simulink model "testControlWithDroneSwarm_r2021b"  (R2021b)
settings: Solver=ode4  StartTime=0.0  StopTime=inf  FixedStep=sample_time_base  RelTol=1e-3
InitFcn:
  | init_condition();
StopFcn:
  | stop_function();
values from neighbouring files (symbols this model uses):
  activate_sim = true    [init_condition.m]
  local_ip = param_simulink.local_ip    [init_condition.m]
  local_ip_sim = param_simulink.local_ip    [init_condition.m]
  number = params.number    [init_condition.m]    (also in visualization.m = size(position0,2))
  number_real = min(param_simulink.number_real,number)    [init_condition.m]    (also in visualization.m = mat_file.number_real)
  number_sim = max(number - number_real,0)    [init_condition.m]
  position0_sim = position0(:,number-number_sim+1:end)    [init_condition.m]
  sample_time_base = 0.0025    [init_condition.m]
  sample_time_control_bottom = sample_time_control_upper    [init_condition.m]
  sample_time_control_upper = params.sample_time_control_upper    [init_condition.m]
  sample_time_motion = sample_time_control_upper    [init_condition.m]    (also in visualization.m = mat_file.sample_time_base)
  target_ip_array = param_simulink.target_ip    [init_condition.m]
  target_ip_array_sim = param_simulink.target_ip(number-number_sim+1:number)    [init_condition.m]
undefined symbols (not defined in the file or in its folder): get_array_slice, map3d_faces, map3d_struct, position0
libraries: aerolibanimutils x1, dspindex x1
settings Model: Creator=huangjialei  LastModifiedBy=Huang Jialei

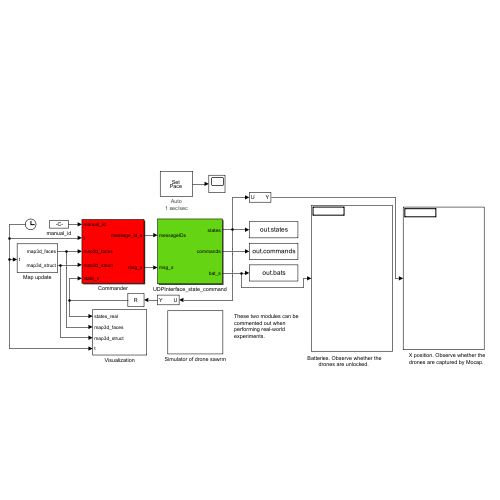
[thumbnail: Simulink's stored preview of the top-level diagram]
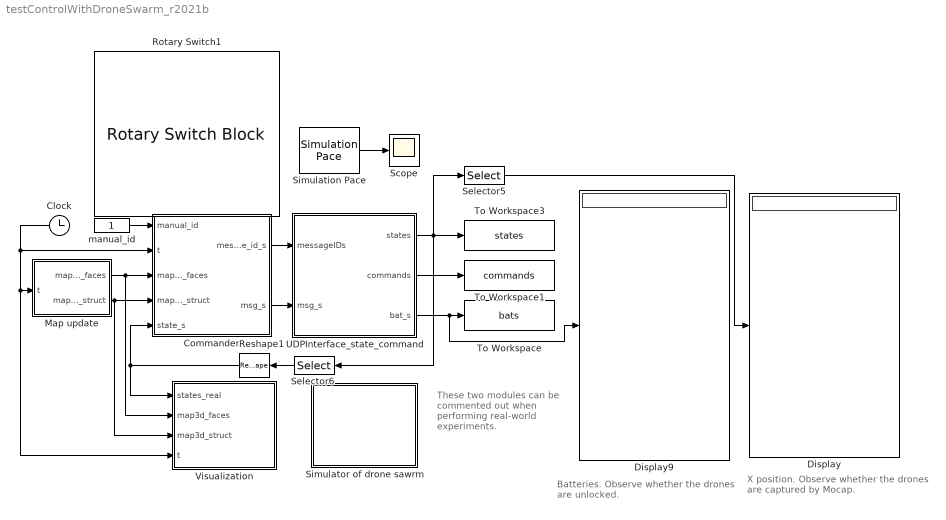
== system testControlWithDroneSwarm_r2021b ==
  note: These two modules can be commented out when performing real-world experiments.
  note: Batteries. Observe whether the drones are unlocked.
  note: X position. Observe whether the drones are captured by Mocap.
  Clock : Clock
  Commander : Subsystem
  Display : Display
  Display9 : Display
  Map update : Subsystem
  Reshape1 : Reshape  OutputDimensionality=Customize  OutputDimensions=[12,number]
  Rotary Switch1 : RotarySwitchBlock
      settings: Values={{'Arming', 'Takeoff', 'Hover', 'Land', 'Alg', 'Test', 'None'}, [1 2 3 4 5 6 1111]}
  Scope : Scope
  Selector5 : Selector  InputPortWidth=17*number  IndexOptions=Index vector (dialog)  Indices=get_array_slice([1,6], number, 17)  OutputSizes=1
  Selector6 : Selector  InputPortWidth=17*number  IndexOptions=Index vector (dialog)  Indices=get_array_slice(6:17, number, 17)  OutputSizes=1
  Simulation Pace : aerolibanimutils/Simulation Pace  SimulationPace=1  SleepMode=Auto  OutputPaceError=on  SampleTime=sample_time_base
  Simulator of drone sawrm : Subsystem
  To Workspace : ToWorkspace  VariableName=bats  SaveFormat=Timeseries  SampleTime=-1
  To Workspace1 : ToWorkspace  VariableName=commands  SaveFormat=Timeseries  SampleTime=-1
  To Workspace3 : ToWorkspace  VariableName=states  SaveFormat=Timeseries  SampleTime=-1
  UDPInterface_state_command : Subsystem
  Visualization : Subsystem
  manual_id : Constant
  wires:
  UDPInterface_state_command/1(states) -> Selector6/1, To Workspace3/1, Selector5/1
  Commander/2(msg_s) -> UDPInterface_state_command/2(msg_s)
  UDPInterface_state_command/2(commands) -> To Workspace1/1
  Commander/1(message_id_s) -> UDPInterface_state_command/1(messageIDs)
  UDPInterface_state_command/3(bat_s) -> Display9/1, To Workspace/1
  Selector5/1 -> Display/1
  manual_id/1 -> Commander/1(manual_id)
  Selector6/1 -> Reshape1/1
  Reshape1/1 -> Commander/5(state_s), Visualization/1(states_real)
  Simulation Pace/1 -> Scope/1
  Map update/1(map3d_faces) -> Visualization/2(map3d_faces), Commander/3(map3d_faces)
  Map update/2(map3d_struct) -> Visualization/3(map3d_struct), Commander/4(map3d_struct)
  Clock/1 -> Visualization/4(t), Map update/1(t), Commander/2(t)

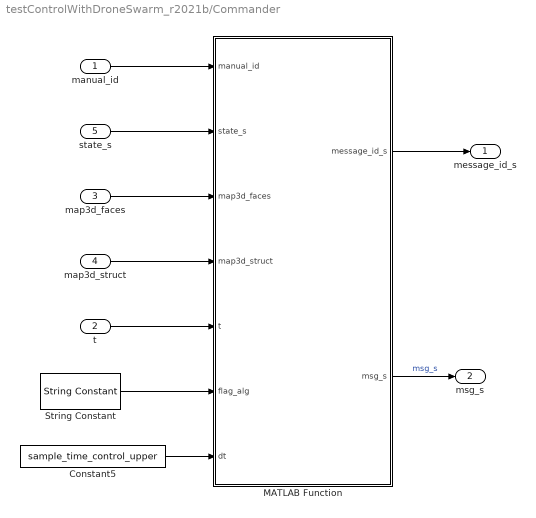
== system testControlWithDroneSwarm_r2021b/Commander ==
  manual_id : Inport
  t : Inport  Port=2
  map3d_faces : Inport  Port=3
  map3d_struct : Inport  Port=4
  state_s : Inport  Port=5
  Constant5 : Constant  Value=sample_time_control_upper
  MATLAB Function : MATLAB Function  TreatAsAtomicUnit=on  SystemSampleTime=sample_time_control_upper
  String Constant : StringConstant  String=flag_alg
  message_id_s : Outport
  msg_s : Outport  Port=2
  wires:
  MATLAB Function/2(msg_s) -> msg_s/1  "msg_s"
  manual_id/1 -> MATLAB Function/1(manual_id)
  t/1 -> MATLAB Function/5(t)
  map3d_faces/1 -> MATLAB Function/3(map3d_faces)
  map3d_struct/1 -> MATLAB Function/4(map3d_struct)
  MATLAB Function/1(message_id_s) -> message_id_s/1
  String Constant/1 -> MATLAB Function/6(flag_alg)
  Constant5/1 -> MATLAB Function/7(dt)
  state_s/1 -> MATLAB Function/2(state_s)

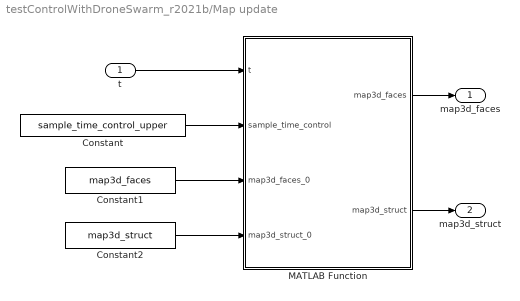
== system testControlWithDroneSwarm_r2021b/Map update ==
  t : Inport
  Constant : Constant  Value=sample_time_control_upper
  Constant1 : Constant  Value=map3d_faces
  Constant2 : Constant  Value=map3d_struct
  MATLAB Function : MATLAB Function  TreatAsAtomicUnit=on  SystemSampleTime=sample_time_control_upper
  map3d_faces : Outport
  map3d_struct : Outport  Port=2
  wires:
  MATLAB Function/1(map3d_faces) -> map3d_faces/1
  MATLAB Function/2(map3d_struct) -> map3d_struct/1
  t/1 -> MATLAB Function/1(t)
  Constant/1 -> MATLAB Function/2(sample_time_control)
  Constant1/1 -> MATLAB Function/3(map3d_faces_0)
  Constant2/1 -> MATLAB Function/4(map3d_struct_0)

== system testControlWithDroneSwarm_r2021b/Simulator of drone sawrm ==
  Constant : Constant  Value=activate_sim
  Simulation : Subsystem
  wires:
  Constant/1 -> Simulation/Enable

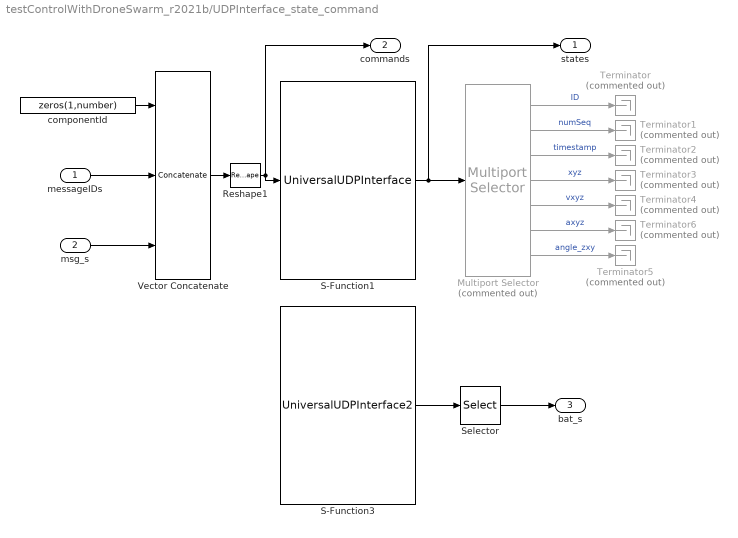
== system testControlWithDroneSwarm_r2021b/UDPInterface_state_command ==
  messageIDs : Inport
  msg_s : Inport  Port=2
  Multiport Selector : dspindex/Multiport Selector  Commented=on  rowsOrCols=Rows  idxCellArray={1:15:15*number,2:15:15*number,3:15:15*number,repmat(4:6,1,number) + reshape(repmat((0:number-1)*15,3,1),1,3*number), repmat(7:9,1,number) + reshape(repmat((0:number-1)*15,3,1),1,3*number), repmat(10:12,1,number) + reshape(repmat((0:number-1)*15,3,1),1,3*number), repmat(13:15,1,number) + reshape(repmat((0:number-1)*15,3,1),1,3*number)}  idxErrMode=Clip Index
  Reshape1 : Reshape
  S-Function1 : S-Function  FunctionName=UniversalUDPInterface  Parameters=sampleTime,number,portTarget,portLocal,ipTarget,ipLocal,flagSend,flagRecv,inputPortWidth,outputPortWidth  SFunctionDeploymentMode=off  EnableBusSupport=off  mask{number=number, ipLocal=local_ip, ipTarget=target_ip_array, portTarget=21000, portLocal=21000, flagSend=on, flagRecv=on, inputPortWidth=6, outputPortWidth=17, sampleTime=sample_time_control_upper}
      mask prompts: number "Number of vehicles"; ipLocal "Local ip"; ipTarget "Target ip"; portTarget "Start port of target"; portLocal "Start port of local"; flagSend "Enable sender"; flagRecv "Enable receiver"; inputPortWidth "Width of input port"; outputPortWidth "Width of output port"; sampleTime "Sample time"
      mask help:
      | input port: componentId, messageId, msgData[0], msgData[1], ...
      | output port: systemId, numSequence, timeStamp,msgData[0], msgData[1], ...
  S-Function3 : S-Function  FunctionName=UniversalUDPInterface2  Parameters=sampleTime,number,portTarget,portLocal,ipTarget,ipLocal,flagSend,flagRecv,inputPortWidth,outputPortWidth  SFunctionDeploymentMode=off  EnableBusSupport=off  mask{number=number, ipLocal=local_ip, ipTarget=target_ip_array, portTarget=22000, portLocal=20000, flagSend=off, flagRecv=on, inputPortWidth=3, outputPortWidth=6, sampleTime=sample_time_control_upper}
      mask prompts: number "Number of vehicles"; ipLocal "Local ip"; ipTarget "Target ip"; portTarget "Start port of target"; portLocal "Start port of local"; flagSend "Enable sender"; flagRecv "Enable receiver"; inputPortWidth "Width of input port"; outputPortWidth "Width of output port"; sampleTime "Sample time"
      mask help:
      | input port: componentId, messageId, msgData[0], msgData[1], ...
      | output port: systemId, numSequence, timeStamp,msgData[0], msgData[1], ...
  Selector : Selector  InputPortWidth=6*number  IndexOptions=Index vector (dialog)  Indices=get_array_slice([1,6], number, 6)  OutputSizes=1
  Terminator{,1..6} (7 alike) : Terminator  Commented=on
  Vector Concatenate : Concatenate  NumInputs=3  Mode=Multidimensional array
  componentId : Constant  Value=zeros(1,number)  VectorParams1D=off
  states : Outport
  commands : Outport  Port=2
  bat_s : Outport  Port=3
  wires:
  Multiport Selector/2 -> Terminator1/1  "numSeq"
  Multiport Selector/5 -> Terminator4/1  "vxyz"
  Vector Concatenate/1 -> Reshape1/1
  Multiport Selector/3 -> Terminator2/1  "timestamp"
  messageIDs/1 -> Vector Concatenate/2
  Reshape1/1 -> S-Function1/1, commands/1
  componentId/1 -> Vector Concatenate/1
  Multiport Selector/4 -> Terminator3/1  "xyz"
  Multiport Selector/1 -> Terminator/1  "ID"
  msg_s/1 -> Vector Concatenate/3
  S-Function3/1 -> Selector/1
  Selector/1 -> bat_s/1
  Multiport Selector/7 -> Terminator5/1  "angle_zxy"
  Multiport Selector/6 -> Terminator6/1  "axyz"
  S-Function1/1 -> states/1, Multiport Selector/1

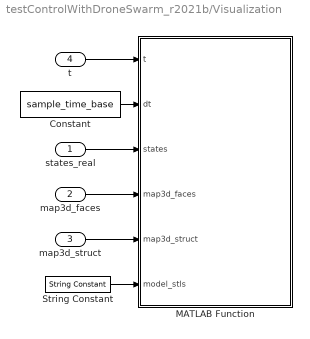
== system testControlWithDroneSwarm_r2021b/Visualization ==
  states_real : Inport
  map3d_faces : Inport  Port=2
  map3d_struct : Inport  Port=3
  t : Inport  Port=4
  Constant : Constant  Value=sample_time_base
  MATLAB Function : MATLAB Function  TreatAsAtomicUnit=on  SystemSampleTime=sample_time_base
  String Constant : StringConstant  String=model_stls
  wires:
  map3d_faces/1 -> MATLAB Function/4(map3d_faces)
  map3d_struct/1 -> MATLAB Function/5(map3d_struct)
  states_real/1 -> MATLAB Function/3(states)
  t/1 -> MATLAB Function/1(t)
  Constant/1 -> MATLAB Function/2(dt)
  String Constant/1 -> MATLAB Function/6(model_stls)

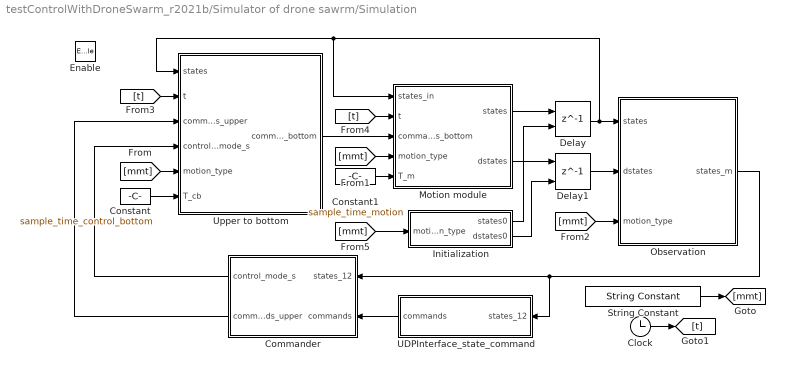
== system testControlWithDroneSwarm_r2021b/Simulator of drone sawrm/Simulation ==
  Enable : EnablePort
  Clock : Clock
  Commander : Subsystem
  Constant : Constant  Value=sample_time_control_bottom
  Constant1 : Constant  Value=sample_time_motion
  Delay : Delay  DelayLength=1  InitialConditionSource=Input port  InitialCondition=0
      settings: InputPortMap=u0,p4
  Delay1 : Delay  DelayLength=1  InitialConditionSource=Input port  InitialCondition=0
      settings: InputPortMap=u0,p4
  Initialization : Subsystem
  Motion module : Subsystem
  Observation : Subsystem
  String Constant : StringConstant  String=motion_model_type
  UDPInterface_state_command : Subsystem
  Upper to bottom : Subsystem
  wires:
  Initialization/2(dstates0) -> Delay1/2
  Delay1/1 -> Observation/2(dstates)
  Motion module/1(states) -> Delay/1
  [mmt] -> Observation/3(motion_type)
  Constant/1 -> Upper to bottom/6(T_cb)
  Upper to bottom/1(commands_bottom) -> Motion module/3(commands_bottom)
  [mmt] -> Motion module/4(motion_type)
  Motion module/2(dstates) -> Delay1/1
  Constant1/1 -> Motion module/5(T_m)
  String Constant/1 -> [mmt]
  UDPInterface_state_command/1(commands) -> Commander/2(commands)
  [mmt] -> Initialization/1(motion_type)
  Commander/1(control_mode_s) -> Upper to bottom/4(control_mode_s)
  Delay/1 -> Observation/1(states), Motion module/1(states_in), Upper to bottom/1(states)
  [t] -> Upper to bottom/2(t)
  Observation/1(states_m) -> Commander/1(states_12), UDPInterface_state_command/1(states_12)
  Initialization/1(states0) -> Delay/2
  [t] -> Motion module/2(t)
  [mmt] -> Upper to bottom/5(motion_type)
  Clock/1 -> [t]
  Commander/2(commands_upper) -> Upper to bottom/3(commands_upper)

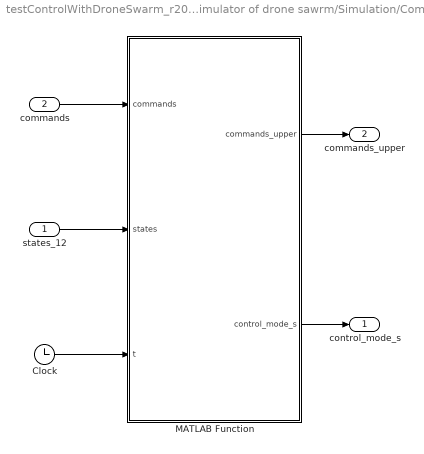
== system testControlWithDroneSwarm_r2021b/Simulator of drone sawrm/Simulation/Commander ==
  states_12 : Inport
  commands : Inport  Port=2
  Clock : Clock
  MATLAB Function : MATLAB Function  TreatAsAtomicUnit=on  SystemSampleTime=sample_time_control_upper
  control_mode_s : Outport
  commands_upper : Outport  Port=2
  wires:
  commands/1 -> MATLAB Function/1(commands)
  states_12/1 -> MATLAB Function/2(states)
  MATLAB Function/1(commands_upper) -> commands_upper/1
  MATLAB Function/2(control_mode_s) -> control_mode_s/1
  Clock/1 -> MATLAB Function/3(t)

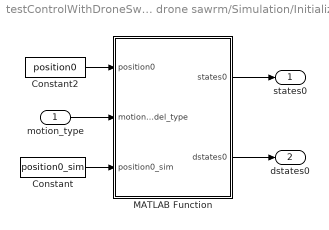
== system testControlWithDroneSwarm_r2021b/Simulator of drone sawrm/Simulation/Initialization ==
  motion_type : Inport
  Constant : Constant  Value=position0_sim
  Constant2 : Constant  Value=position0
  MATLAB Function : MATLAB Function  TreatAsAtomicUnit=on
  states0 : Outport
  dstates0 : Outport  Port=2
  wires:
  MATLAB Function/1(states0) -> states0/1
  Constant2/1 -> MATLAB Function/1(position0)
  motion_type/1 -> MATLAB Function/2(motion_model_type)
  MATLAB Function/2(dstates0) -> dstates0/1
  Constant/1 -> MATLAB Function/3(position0_sim)

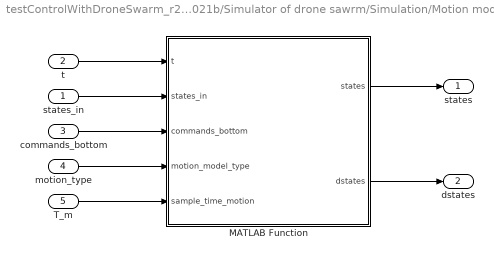
== system testControlWithDroneSwarm_r2021b/Simulator of drone sawrm/Simulation/Motion module ==
  states_in : Inport
  t : Inport  Port=2
  commands_bottom : Inport  Port=3
  motion_type : Inport  Port=4
  T_m : Inport  Port=5
  MATLAB Function : MATLAB Function  TreatAsAtomicUnit=on  SystemSampleTime=sample_time_motion
  states : Outport
  dstates : Outport  Port=2
  wires:
  t/1 -> MATLAB Function/1(t)
  MATLAB Function/1(states) -> states/1
  MATLAB Function/2(dstates) -> dstates/1
  states_in/1 -> MATLAB Function/2(states_in)
  commands_bottom/1 -> MATLAB Function/3(commands_bottom)
  motion_type/1 -> MATLAB Function/4(motion_model_type)
  T_m/1 -> MATLAB Function/5(sample_time_motion)

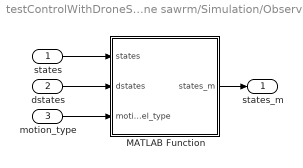
== system testControlWithDroneSwarm_r2021b/Simulator of drone sawrm/Simulation/Observation ==
  states : Inport
  dstates : Inport  Port=2
  motion_type : Inport  Port=3
  MATLAB Function : MATLAB Function  TreatAsAtomicUnit=on
  states_m : Outport
  wires:
  MATLAB Function/1(states_m) -> states_m/1
  states/1 -> MATLAB Function/1(states)
  dstates/1 -> MATLAB Function/2(dstates)
  motion_type/1 -> MATLAB Function/3(motion_model_type)

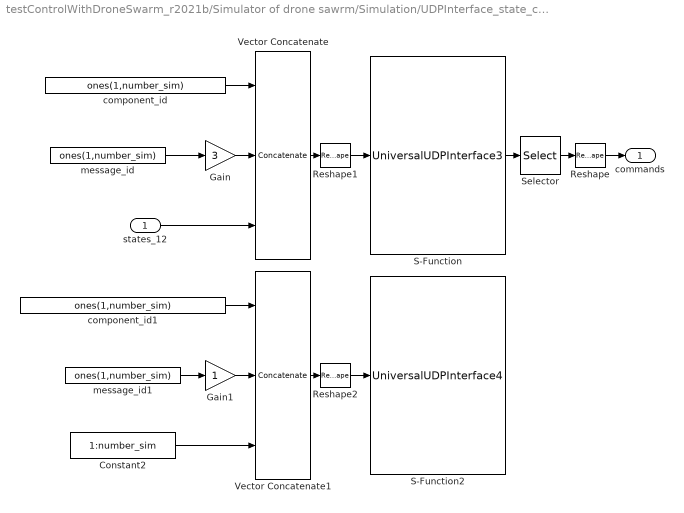
== system testControlWithDroneSwarm_r2021b/Simulator of drone sawrm/Simulation/UDPInterface_state_command ==
  states_12 : Inport
  Constant2 : Constant  Value=1:number_sim  VectorParams1D=off
  Gain : Gain  Gain=3
  Gain1 : Gain
  Reshape : Reshape  OutputDimensionality=Customize  OutputDimensions=[6,number_sim]
  Reshape1 : Reshape
  Reshape2 : Reshape
  S-Function : S-Function  FunctionName=UniversalUDPInterface3  Parameters=sampleTime,number,portTarget,portLocal,ipTarget,ipLocal,flagSend,flagRecv,inputPortWidth,outputPortWidth  SFunctionDeploymentMode=off  EnableBusSupport=off  mask{number=number_sim, ipLocal=local_ip_sim, ipTarget=target_ip_array_sim, portTarget=20999+number_real*2, portLocal=21001+number_real*2, flagSend=on, flagRecv=on, inputPortWidth=14, outputPortWidth=9, sampleTime=sample_time_control_upper}
      mask prompts: number "Number of vehicles"; ipLocal "Local ip"; ipTarget "Target ip"; portTarget "Start port of target"; portLocal "Start port of local"; flagSend "Enable sender"; flagRecv "Enable receiver"; inputPortWidth "Width of input port"; outputPortWidth "Width of output port"; sampleTime "Sample time"
      mask help:
      | input port: componentId, messageId, msgData[0], msgData[1], ...
      | output port: systemId, numSequence, timeStamp,msgData[0], msgData[1], ...
  S-Function2 : S-Function  FunctionName=UniversalUDPInterface4  Parameters=sampleTime,number,portTarget,portLocal,ipTarget,ipLocal,flagSend,flagRecv,inputPortWidth,outputPortWidth  SFunctionDeploymentMode=off  EnableBusSupport=off  mask{number=number_sim, ipLocal=local_ip_sim, ipTarget=target_ip_array_sim, portTarget=19999+number_real*2, portLocal=22001+number_real*2, flagSend=on, flagRecv=off, inputPortWidth=3, outputPortWidth=9, sampleTime=sample_time_control_upper}
      mask prompts: number "Number of vehicles"; ipLocal "Local ip"; ipTarget "Target ip"; portTarget "Start port of target"; portLocal "Start port of local"; flagSend "Enable sender"; flagRecv "Enable receiver"; inputPortWidth "Width of input port"; outputPortWidth "Width of output port"; sampleTime "Sample time"
      mask help:
      | input port: componentId, messageId, msgData[0], msgData[1], ...
      | output port: systemId, numSequence, timeStamp,msgData[0], msgData[1], ...
  Selector : Selector  InputPortWidth=9*number_sim  IndexOptions=Index vector (dialog)  Indices=get_array_slice(4:9, number_sim, 9)  OutputSizes=1
  Vector Concatenate : Concatenate  NumInputs=3  Mode=Multidimensional array
  Vector Concatenate1 : Concatenate  NumInputs=3  Mode=Multidimensional array
  component_id : Constant  Value=ones(1,number_sim)  VectorParams1D=off
  component_id1 : Constant  Value=ones(1,number_sim)  VectorParams1D=off
  message_id : Constant  Value=ones(1,number_sim)  VectorParams1D=off
  message_id1 : Constant  Value=ones(1,number_sim)  VectorParams1D=off
  commands : Outport
  wires:
  Reshape/1 -> commands/1
  Selector/1 -> Reshape/1
  states_12/1 -> Vector Concatenate/3
  Vector Concatenate1/1 -> Reshape2/1
  Reshape2/1 -> S-Function2/1
  component_id1/1 -> Vector Concatenate1/1
  Constant2/1 -> Vector Concatenate1/3
  message_id1/1 -> Gain1/1
  Gain1/1 -> Vector Concatenate1/2
  S-Function/1 -> Selector/1
  Gain/1 -> Vector Concatenate/2
  message_id/1 -> Gain/1
  component_id/1 -> Vector Concatenate/1
  Reshape1/1 -> S-Function/1
  Vector Concatenate/1 -> Reshape1/1

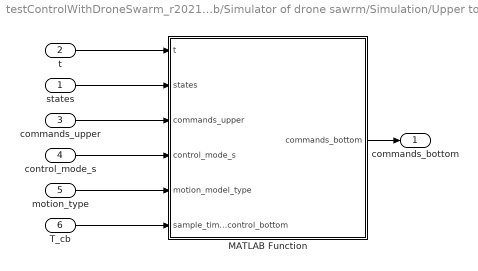
== system testControlWithDroneSwarm_r2021b/Simulator of drone sawrm/Simulation/Upper to bottom ==
  states : Inport
  t : Inport  Port=2
  commands_upper : Inport  Port=3
  control_mode_s : Inport  Port=4
  motion_type : Inport  Port=5
  T_cb : Inport  Port=6
  MATLAB Function : MATLAB Function  TreatAsAtomicUnit=on  SystemSampleTime=sample_time_control_bottom
  commands_bottom : Outport
  wires:
  MATLAB Function/1(commands_bottom) -> commands_bottom/1
  states/1 -> MATLAB Function/2(states)
  t/1 -> MATLAB Function/1(t)
  commands_upper/1 -> MATLAB Function/3(commands_upper)
  control_mode_s/1 -> MATLAB Function/4(control_mode_s)
  motion_type/1 -> MATLAB Function/5(motion_model_type)
  T_cb/1 -> MATLAB Function/6(sample_time_control_bottom)

== matlab function testControlWithDroneSwarm_r2021b/Simulator of drone sawrm/Simulation/Initialization/MATLAB Function ==
  data: position0 input; states0 output; motion_model_type input; dstates0 output; position0_sim input
function [states0,dstates0] = fcn(position0, motion_model_type, position0_sim)

number_sim = size(position0_sim,2);
number = size(position0,2);
states0 = zeros(17,number_sim);
dstates0 = zeros(17,number_sim);

number_real = number - number_sim;

[states,dstates] = initialize_states(position0, motion_model_type);


temp = size(states,1);
states0(1:temp,:) = states(:,number_real+1:end);
temp = size(dstates,1);
dstates0(1:temp,:) = dstates(:,number_real+1:end);

== matlab function testControlWithDroneSwarm_r2021b/Commander/MATLAB Function ==
  data: message_id_s output; manual_id input; state_s input; msg_s output; map3d_faces input; map3d_struct input; t input; flag_alg input; dt input
function [message_id_s, msg_s] = swarm_algorithm(manual_id,state_s, map3d_faces, map3d_struct, t, flag_alg, dt)

number_all = size(state_s,2);
msg_s = zeros(4,number_all);
message_id_s = zeros(1,number_all);

% If the agent is not captured by mocap, its states are all 0. 
is_running = sum(abs(state_s(1:6,:)),1) > 0.001;

%%
% Value of rotary switch
manual_arming = 1;
manual_takeoff = 2;
manual_hover = 3;
manual_land = 4;
manual_alg = 5;
manual_test = 6;
% External control mode
Arming_type = 1;
Takeoff_type = 2;
Hover_type = 3;
Land_type = 4;
Position_control_type = 5;
Velocity_control_type = 6;
Velocity_horizontal_control_type = 7;

% coder.extrinsic('swarm_module_generate_desire');
% coder.extrinsic('py.sorted');
% disp(py.sorted([2,3,1]));
%
h_takeoff = 0.7;
h_land = 0.0;
switch manual_id
    case manual_arming
        message_id_s = Arming_type * ones(1,number_all);
        msg_s = zeros(4,number_all);
    case manual_takeoff
        message_id_s = Takeoff_type * ones(1,number_all);
        msg_s = zeros(4,number_all);
        msg_s(1,:) = h_takeoff;
    case manual_hover
        message_id_s = Hover_type * ones(1,number_all);
        msg_s = zeros(4,number_all);
    case manual_land
        message_id_s = Land_type * ones(1,number_all);
        msg_s = zeros(4,number_all);
        msg_s(1,:) = h_land;
    case manual_alg
        id_is_running = find(is_running);
%         vel_desired = zeros(2, length(id_is_running));
        number_isr = length(id_is_running);
        pos_desired_s_isr = zeros(4,number_isr);
        vel_desired_s_isr = zeros(4,number_isr);

        if sensor_env_module_get_activate()
            motion_model_type = 'quadcopter'; %%%%%%%%%%%%%%%%%%%%
            sensor_data_s = sensor_env_module_get_data_all(state_s(:,id_is_running), motion_model_type, map3d_faces);
        else
            sensor_data_s = [];
        end
        [command_upper_s_isr,control_mode_s_u_isr] = ...
            swarm_module_generate_desire(t, state_s(:,id_is_running), flag_alg, dt, sensor_data_s, map3d_struct);
        
        pos_desired_s_isr(:) = command_upper_s_isr(1:4,1:number_isr);
        vel_desired_s_isr(:) = command_upper_s_isr(5:8,1:number_isr);
  
        message_id_s(id_is_running) = control_mode_s_u_isr;
        control_mode_unique = unique(control_mode_s_u_isr);
        
        for c = 1:length(control_mode_unique)
            control_mode = control_mode_unique(c);
            id_selected_isr = find(control_mode_s_u_isr==control_mode);
            msg_s_isr = zeros(4,length(id_selected_isr));
            switch control_mode
                case Takeoff_type
                    message_id_s = Takeoff_type * ones(1,number_all);
                    msg_s_isr(1,:) = pos_desired_s_isr(3,id_selected_isr);
                case Land_type
                    message_id_s = Land_type * ones(1,number_all);
                    msg_s_isr(1,:) = pos_desired_s_isr(3,id_selected_isr);
                case Hover_type
                    message_id_s = Hover_type * ones(1,number_all);
                case Position_control_type
                    message_id_s = Land_type * ones(1,number_all);
                    msg_s_isr(:,:) = pos_desired_s_isr(:,id_selected_isr);
                case Velocity_control_type
                    message_id_s = Velocity_control_type * ones(1,number_all);
                    msg_s_isr(:,:) = vel_desired_s_isr(:,id_selected_isr);
                case Velocity_horizontal_control_type 
                    message_id_s = Velocity_horizontal_control_type * ones(1,number_all);
                    msg_s_isr([1,2,4],:) = vel_desired_s_isr([1,2,4],id_selected_isr);
                    msg_s_isr(3,:) = pos_desired_s_isr(3,id_selected_isr);
            end
            id_selected = id_is_running(id_selected_isr);
            msg_s(:,id_selected) = msg_s_isr;
        end
    case manual_test
        xyz_s = state_s(1:3,:);
        vxyz_s = state_s(4:6,:);
        id_is_running = find(is_running);
        num_is_runnning = length(id_is_running);
        xyz_s_is_running = xyz_s(:,is_running);
        vxyz_s_is_running = vxyz_s(:,is_running);
        velDesired = zeros(3,num_is_runnning);
        % Params
        v_flock = 0.4;
        z_d = 0.7;
        r_rep = 1.0;
        p_rep = 1.0;
        v_wall_0 = 0.4;
        x_range_wall = [-1.5,1.5];
        y_range_wall = [-1.5,1.5];
        v_max = 0.4;
        % =============Behaviors=============
        % Alignment
        v_vist = mean(vxyz_s_is_running(1:2,:),2);
        v_vist_norm = norm(v_vist);
        if v_vist_norm>0
            v_vist = v_vist/v_vist_norm * v_flock;
        else
            v_vist = rand(2,1);
            v_vist = v_vist/norm(v_vist) * v_flock;
        end
        % Repulsion
        v_rep = zeros(2,num_is_runnning);
        x_ij = repmat(xyz_s_is_running(1,:),num_is_runnning,1) -...
            repmat(xyz_s_is_running(1,:)',1,num_is_runnning);
        y_ij = repmat(xyz_s_is_running(2,:),num_is_runnning,1) -...
            repmat(xyz_s_is_running(2,:)',1,num_is_runnning);
        d_ij = sqrt(x_ij.^2 + y_ij.^2);
        d_ij(1:num_is_runnning+1:num_is_runnning^2) = r_rep*100;
        in_rep = double(d_ij < r_rep);
        v_rep(1,:) = p_rep*sum( (r_rep - d_ij).*x_ij./d_ij.*in_rep ,1);
        v_rep(2,:) = p_rep*sum( (r_rep - d_ij).*y_ij./d_ij.*in_rep ,1);
        % Wall avoidance
        v_wall = zeros(2,num_is_runnning);
        v_wall(1,:) = double(xyz_s_is_running(1,:) < x_range_wall(1)) * 1.0 + ...
            double(xyz_s_is_running(1,:) > x_range_wall(2)) * (-1.0);
        v_wall(2,:) = double(xyz_s_is_running(2,:) < y_range_wall(1)) * 1.0 + ...
            double(xyz_s_is_running(2,:) > y_range_wall(2)) * (-1.0);
        v_wall_norm = sqrt(sum(v_wall.^2,1));
        v_wall_norm(v_wall_norm==0) = 10;
        v_wall = v_wall_0*v_wall./v_wall_norm;

        % Combination
        velDesired(1:2,:) = repmat(v_vist,1,num_is_runnning) + v_rep + v_wall;
        velDesired_norm = sqrt(sum(velDesired(1:2,:).^2,1));
        temp = find(velDesired_norm>v_max);
        if ~isempty(temp)
            velDesired(1:2,temp) = v_max*velDesired(1:2,temp)./velDesired_norm(temp);
        end
        %
%         message_id_s(id_is_running) = Velocity_horizontal_control_type;
%         msg_s(1,id_is_running) = velDesired(1,:);
%         msg_s(2,id_is_running) = velDesired(2,:);
%         msg_s(3,id_is_running) = z_d; % z_d
%         msg_s(4,id_is_running) = 0.0; % yaw_rate_d
        %
        message_id_s(id_is_running) = Velocity_control_type;
        msg_s(1,id_is_running) = velDesired(1,:);
        msg_s(2,id_is_running) = velDesired(2,:);
        msg_s(3,id_is_running) = 0.1*sin(t); % vz_d
        msg_s(4,id_is_running) = 0.0; % yaw_rate_d
    otherwise

end

== matlab function testControlWithDroneSwarm_r2021b/Map update/MATLAB Function ==
  data: t input; map3d_faces output; sample_time_control input; map3d_faces_0 input; map3d_struct_0 input; map3d_struct output
function [map3d_faces,map3d_struct] = fcn(t, sample_time_control,map3d_faces_0, map3d_struct_0)

persistent map3d_faces_new map3d_struct_new
if isempty(map3d_faces_new) || t==0
    map3d_faces_new = map3d_faces_0;
    map3d_struct_new = map3d_struct_0;
end


[map3d_faces_new,map3d_struct_new] = map_module_update_map3d(t, sample_time_control,map3d_faces_new, map3d_struct_new);

map3d_faces = map3d_faces_new;
map3d_struct = map3d_struct_new;

== matlab function testControlWithDroneSwarm_r2021b/Visualization/MATLAB Function ==
  data: t input; dt input; states input; map3d_faces input; map3d_struct input; model_stls input
function fcn(t, dt, states, map3d_faces, map3d_struct, model_stls)
coder.extrinsic('draw_environment');
coder.extrinsic('adjust_figure_axis');
coder.extrinsic('num2str');
coder.extrinsic('draw_body');
coder.extrinsic('split');

persistent f_1 a_1

[activate_plot,...
    time_interval_plot,...
    activate_trajectory,...
    follow_agent,...
    activate_save_figure,...
    activate_save_video,...
    dim_visual,...
    time_interval_trajectory,...
    video_speed] = visual_module_parameters();

if ~activate_plot
    return
end

if t == 0 || isempty(f_1) || isempty(a_1)
    start_and_end = 1;
    f_1 = figure;
    a_1 = gca;
    hold(a_1,'on'); grid(a_1,'on'); box(a_1,'on')
    axis(a_1,'equal')
    xlabel(a_1,'X Position (m)');
    ylabel(a_1,'Y Position (m)');
    if dim_visual == 3
        zlabel(a_1,'Z Position (m)');
        view(a_1,[-45,30]);
    end
    title(a_1,['Elapsed time ',num2str(t,"%.2f"),' s'])
    [x_range,y_range,z_range] = get_range(states, map3d_faces);
    xlim(a_1,x_range);
    ylim(a_1,y_range);
    zlim(a_1,z_range);
else
    start_and_end = 0;
end

flag_motion_model = 1;
if visual_module_get_activate(dt,t,start_and_end)
    draw_environment(a_1, map3d_faces, map3d_struct, split(model_stls), dim_visual);

    num = size(states,2);
    len_arm = 0.1;
    color_s_bodies = zeros(3,num);
    draw_body(a_1, states, dim_visual, flag_motion_model, len_arm, color_s_bodies);
    title(a_1,['Elapsed time ',num2str(t,"%.2f"),' s'])
    [x_range,y_range,z_range] = get_range(states, map3d_faces);
    % xlim(a_1,x_range);
    % ylim(a_1,y_range);
    % zlim(a_1,z_range);
end

    function [x_range,y_range,z_range] = get_range(states, map3d_faces)
        if ~isempty(map3d_faces)
            x_range = [min(map3d_faces(1:3:9,:),[],'all'),max(map3d_faces(1:3:9,:),[],'all')];
            y_range = [min(map3d_faces(2:3:9,:),[],'all'),max(map3d_faces(2:3:9,:),[],'all')];
            z_range = [min(map3d_faces(3:3:9,:),[],'all'),max(map3d_faces(3:3:9,:),[],'all')];
        else
            x_range = [min(states(1,:)),max(states(1,:))];
            y_range = [min(states(2,:)),max(states(2,:))];
            z_range = [min(states(3,:)),max(states(3,:))];
        end
        if x_range(2) - x_range(1) <=0
            x_range = [0,1];
        end
        if y_range(2) - y_range(1) <=0
            y_range = [0,1];
        end
        if z_range(2) - z_range(1) <=0
            z_range = [0,1];
        end
    end
end

== matlab function testControlWithDroneSwarm_r2021b/Simulator of drone sawrm/Simulation/Commander/MATLAB Function ==
  settings: updateMethod=DISCRETE
  data: commands input; commands_upper output; states input; t input; control_mode_s output
function [commands_upper, control_mode_s] = commander(commands, states,t)
persistent states_save  message_Ids_former t_start_Circle t_trigger v_save vx_save vy_save
number = size(states,2);
if isempty(states_save) || t < 0.1
    states_save = states;
    message_Ids_former = zeros(1,number)-1;
end
xyz_s = states(1:3,:);
% vxyz_s = states(4:6,:);
% axyz_s = states(7:9,:);
yrp_s = states(10:12,:);

xyzYaw_ds = [xyz_s;yrp_s(1,:)];
vxyzYr_ds_fw = zeros(4,number);
axyz_ds_fw   = zeros(4,number);



component_ids = commands(1,:);
message_ids = commands(2,:);
msgs = commands(3:6,:);

COMMAND_TYPE = 0;

Arming = 1;
Takeoff = 2;
Hover = 3;
Land = 4;
Position_control = 5;
Velocity_control = 6;
Velocity_horizontal_control = 7;
Acceleration_control = 8;

control_mode_s = message_ids;

for id = 1:number
    component_id = component_ids(id);
    if component_id == COMMAND_TYPE
        message_id = message_ids(id);
        message_id_former = message_Ids_former(id);
        msg = msgs(:,id);
        
        switch message_id
            case Arming
                if message_id_former ~= message_id
                    fprintf("UAV %d armed.\n",int16(id));
                    states_save(:,id) = states(:,id);
                end
                xyzYaw_ds(:,id) = states_save([1,2,3,10],id);
                control_mode_s(id) = Position_control;
            case Takeoff
                if message_id_former ~= message_id
%                     str = sprintf("UAV %d takeoff.",id);
%                     disp(str);
%                     disp(str);
                    fprintf("UAV %d takeoff.\n",int16(id));
                    states_save(:,id) = states(:,id);
                end
                xyzYaw_ds(:,id) = states_save([1,2,3,10],id);
                xyzYaw_ds(3,id) = msg(1);
                control_mode_s(id) = Position_control;
            case Hover
                if message_id_former ~= message_id
%                     disp(['UAV ',num2str(id),' hover.']);
                    states_save(:,id) = states(:,id);
                end
                xyzYaw_ds(:,id) = states_save([1,2,3,10],id);
                control_mode_s(id) = Position_control;
            case Land
                if message_id_former ~= message_id
%                     disp(['UAV ',num2str(id),' land.']);
                    states_save(:,id) = states(:,id);
                end
                xyzYaw_ds(:,id) = states_save([1,2,3,10],id);
                xyzYaw_ds(3,id) = msg(1);
                control_mode_s(id) = Position_control;
            case Position_control
                if message_id_former ~= message_id
%                     disp(['UAV ',num2str(id),' position control.']);
                end
                xyzYaw_ds(:,id) = msg;
            case Velocity_control
                if message_id_former ~= message_id
%                     disp(['UAV ',num2str(id),' velocity control.']);
                end
                vxyzYr_ds_fw(:,id) = msg;
            case Velocity_horizontal_control
                if message_id_former ~= message_id
%                     disp(['UAV ',num2str(id),' velocity horizontal control.']);
                end
                vxyzYr_ds_fw([1,2,4],id) = msg([1,2,4]);
                xyzYaw_ds(3,id) = msg(3);
            case Acceleration_control
                if message_id_former ~= message_id
%                     disp(['UAV ',num2str(id),' acceleration control.']);
                end
                axyz_ds_fw(1:3,id) = msg(1:3);
            otherwise
                if message_id_former ~= message_id
%                     disp(['UAV ',num2str(id),' hover.']);
                    states_save(:,id) = states(:,id);
                end
                xyzYaw_ds(:,id) = states_save([1,2,3,10],id);
                control_mode_s(id) = Position_control;
        end
        message_Ids_former(id) = message_id;
    end
end


commands_upper = [xyzYaw_ds;vxyzYr_ds_fw;axyz_ds_fw];

== matlab function testControlWithDroneSwarm_r2021b/Simulator of drone sawrm/Simulation/Motion module/MATLAB Function ==
  data: t input; states output; states_in input; commands_bottom input; motion_model_type input; sample_time_motion input; dstates output
function [states, dstates] = fcn(t, states_in, commands_bottom, motion_model_type, sample_time_motion)

number = size(states_in,2);
% Dynamics and kinematics simulation
states = zeros(17,number);
dstates = zeros(17,number);


[states_, dstates_] = motion_module_update_dynamics(t, states_in,commands_bottom,...
    motion_model_type, sample_time_motion);

temp = size(states_,1);
states(1:temp,:) = states_;
dstates(1:temp,:) = dstates_;

== matlab function testControlWithDroneSwarm_r2021b/Simulator of drone sawrm/Simulation/Upper to bottom/MATLAB Function ==
  data: t input; commands_bottom output; states input; commands_upper input; control_mode_s input; motion_model_type input; sample_time_control_bottom input
function commands_bottom = fcn(t, states, commands_upper, control_mode_s, motion_model_type, sample_time_control_bottom)

 % Bottom control
number = size(states,2);
commands_bottom = zeros(4,number);

 commands_bottom_ = motion_module_bottom_control(t, states, commands_upper,...
     control_mode_s, motion_model_type, sample_time_control_bottom);

 temp = size(commands_bottom_,1);
 commands_bottom(1:temp,:) = commands_bottom_;

== matlab function testControlWithDroneSwarm_r2021b/Simulator of drone sawrm/Simulation/Observation/MATLAB Function ==
  data: states input; dstates input; states_m output; motion_model_type input
function states_m = fcn(states,dstates,motion_model_type)

number = size(states,2);
states_m = zeros(12,number);

% Observation
states_ob = motion_module_observation(states,dstates,motion_model_type);

% Add noise to states_ob
states_m_ = noise_module_add_noise(states_ob);

temp = size(states_m_,1);


states_m(1:temp,:) = states_m_;
